simulink model "Exercitiul1"  (R2016a)
settings: Solver=VariableStepAuto  StartTime=0.0  StopTime=17280  RelTol=1e-3
undefined symbols (not defined in the file): m, n
settings Model: Creator=Cristina  LastModifiedBy=Cristina

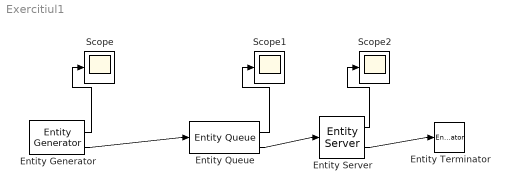
== system Exercitiul1 ==
  Entity Generator : EntityGenerator  OutputPortMessageModes=n,m  TimeSource=MATLAB action  IntergenerationTimeAction=|  NumberEntitiesDeparted=on  EntityType=Structured  EntityTypeName=Entity
      | persistent init
      | if (isempty(init))
      |     rng(1437);
      |     init = true;
      | end
      | dt = 12 + rand * 12;
      settings: OutputPortMap=o0,o3
  Entity Queue : EntityQueue  InputPortMessageModes=m  OutputPortMessageModes=n,m  Capacity=100  NumberEntitiesInBlock=on
      settings: OutputPortMap=o1,o5
  Entity Server : EntityServer  InputPortMessageModes=m  OutputPortMessageModes=n,m  Capacity=1  ServiceTimeSource=MATLAB action  ServiceTimeAction=|  NumberEntitiesDeparted=on
      | persistent init
      | if (isempty(init))
      |     rng(1437);
      |     init = true;
      | end
      | dt = 12 + rand * 8;
      settings: OutputPortMap=o0,o9
  Entity Terminator : EntityTerminator  InputPortMessageModes=m
  Scope : Scope
  Scope1 : Scope
  Scope2 : Scope
  wires:
  Entity Generator/2 -> Entity Queue/1
  Entity Queue/2 -> Entity Server/1
  Entity Server/2 -> Entity Terminator/1
  Entity Generator/1 -> Scope/1
  Entity Server/1 -> Scope2/1
  Entity Queue/1 -> Scope1/1
